simulink model "pd_control"  (R2023b)
settings: Solver=VariableStepAuto  StartTime=0.0  StopTime=10.0  RelTol=1e-3
values from neighbouring files (symbols this model uses):
  a = [x;y;z]    [generate_trajectory.m]    (also in init.m = 1)
  A = 0.1    [generate_trajectory.m]    (also in get_FrictionTorque.m = fp(1,:); init.m = 0.4)
  B = 0.1    [generate_trajectory.m]    (also in init.m = 0.4)
  b = 2    [generate_trajectory.m]    (also in init.m)
  d = pi/2    (= 1.57079632679)    [init.m]
  dq0 = [0.0 ; 0.0; 0.0 ; 0.0; 0.0 ; 0.0; 0.0]    [init.m]
  Kp = 10*eye(7)    [init.m]
  Kv = 10*eye(7)    [init.m]
  Lambda_IK = 10*eye(3)    [init.m]
  lev_mar = false    [init.m]
  mu_0 = 1e-2    (= 0.01)    [init.m]
  p0 = [0.85; 0.85; 0.85]    [init.m]
  q0 = [0 0 0 0 0 0 0]    [FRANKA_model.m]    (also in generate_trajectory.m = [0 pi/3 0 pi/6 0 0 0]; init.m = [0.25 ; 0.25; 0.25 ; 0.25; 0.25 ; 0.25; 0.25])
  rel_err = 0.0    (= 0)    [init.m]
libraries: robotmaniplib x1
settings Model: Creator=franc  LastModifiedBy=franc

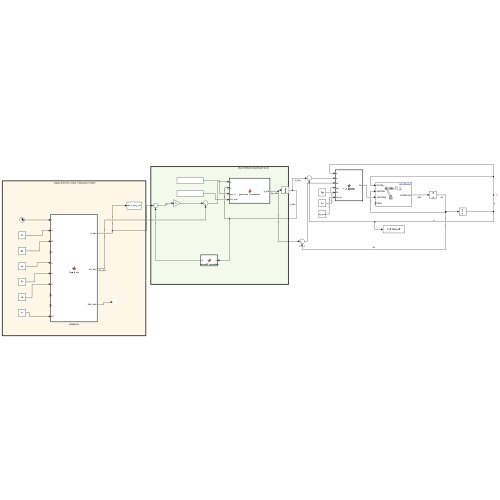
[thumbnail: Simulink's stored preview of the top-level diagram]
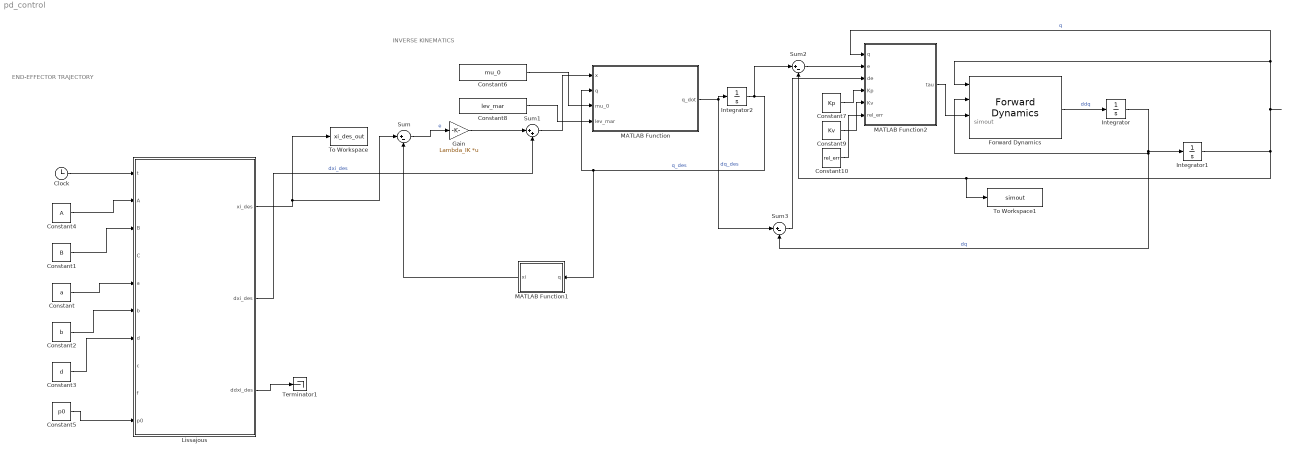
== system pd_control ==
  note: simout
  note: END-EFFECTOR TRAJECTORY
  note: INVERSE KINEMATICS
  Clock : Clock
  Constant : Constant  Value=a
  Constant1 : Constant  Value=B
  Constant10 : Constant  Value=rel_err
  Constant2 : Constant  Value=b
  Constant3 : Constant  Value=d
  Constant4 : Constant  Value=A
  Constant5 : Constant  Value=p0
  Constant6 : Constant  Value=mu_0
  Constant7 : Constant  Value=Kp  VectorParams1D=off
  Constant8 : Constant  Value=lev_mar
  Constant9 : Constant  Value=Kv  VectorParams1D=off
  Forward Dynamics : robotmaniplib/Forward Dynamics  RigidBodyTree=robotModel  SimulateUsing=Interpreted execution
  Gain : Gain  Gain=Lambda_IK  Multiplication=Matrix(K*u)
  Integrator : Integrator  InitialCondition=dq0
  Integrator1 : Integrator  InitialCondition=q0
  Integrator2 : Integrator  InitialCondition=q0
  Lissajous : MATLAB Function  TreatAsAtomicUnit=on
  MATLAB Function : MATLAB Function  TreatAsAtomicUnit=on
  MATLAB Function1 : MATLAB Function  TreatAsAtomicUnit=on
  MATLAB Function2 : MATLAB Function  TreatAsAtomicUnit=on
  Sum : Sum  Inputs=|+-
  Sum1 : Sum  Inputs=|++
  Sum2 : Sum  Inputs=|+-
  Sum3 : Sum  Inputs=|+-
  Terminator1 : Terminator
  To Workspace : ToWorkspace  VariableName=xi_des_out  SaveFormat=Timeseries  SampleTime=-1
  To Workspace1 : ToWorkspace  VariableName=simout  SaveFormat=Timeseries  SampleTime=-1
  wires:
  Forward Dynamics/1 -> Integrator/1  "ddq"
  Integrator/1 -> Sum3/2, Forward Dynamics/2, Integrator1/1  "dq"
  Integrator1/1 -> MATLAB Function2/1(q), Forward Dynamics/1, To Workspace1/1, Sum2/2  "q"
  MATLAB Function/1(q_dot) -> Integrator2/1, Sum3/1  "dq_des"
  Integrator2/1 -> Sum2/1, MATLAB Function1/1(q), MATLAB Function/2(q)  "q_des"
  Constant3/1 -> Lissajous/7(d)
  Constant5/1 -> Lissajous/10(p0)
  Lissajous/1(xi_des) -> To Workspace/1, Sum/1
  Clock/1 -> Lissajous/1(t)
  Constant4/1 -> Lissajous/2(A)
  Constant/1 -> Lissajous/5(a)
  Constant1/1 -> Lissajous/3(B)
  Constant2/1 -> Lissajous/6(b)
  Lissajous/3(ddxi_des) -> Terminator1/1
  MATLAB Function1/1(xi) -> Sum/2
  Gain/1 -> Sum1/1
  Sum/1 -> Gain/1  "e"
  Sum1/1 -> MATLAB Function/1(x)
  Constant6/1 -> MATLAB Function/3(mu_0)
  Constant8/1 -> MATLAB Function/4(lev_mar)
  Lissajous/2(dxi_des) -> Sum1/2  "dxi_des"
  Sum2/1 -> MATLAB Function2/2(e)
  Sum3/1 -> MATLAB Function2/3(de)
  Constant7/1 -> MATLAB Function2/4(Kp)
  Constant9/1 -> MATLAB Function2/5(Kv)
  MATLAB Function2/1(tau) -> Forward Dynamics/3
  Constant10/1 -> MATLAB Function2/6(rel_err)

== matlab function pd_control/MATLAB Function1 ==
  data: q input; xi output
function xi = forwardKinematics(q)
q1 = q(1);
q2 = q(2);
q3 = q(3);
q4 = q(4);
q5 = q(5);
q6 = q(6);
q7 = q(7);
T01r = [cos(q1), -sin(q1), 0;
       sin(q1) , cos(q1), 0;
        0, 0, 1];
T12r = [cos(q2), -sin(q2), 0;
       sin(q2) , cos(q2), 0;
        0, 0, 1] * [1, 0, 0;
            0, cos(-pi/2), -sin(-pi/2);
            0, sin(-pi/2), cos(-pi/2)]; 
T23r = [cos(q3), -sin(q3), 0;
       sin(q3) , cos(q3), 0;
        0, 0, 1] * [1, 0, 0;
            0, cos(pi/2), -sin(pi/2);
            0, sin(pi/2), cos(pi/2)]; 

T23t = [0 0 0.42]';


T34r = [cos(q4), -sin(q4), 0;
       sin(q4) , cos(q4), 0;
        0, 0, 1] * [1, 0, 0;
            0, cos(pi/2), -sin(pi/2);
            0, sin(pi/2), cos(pi/2)]; 
T45r = [cos(q5), -sin(q5), 0;
       sin(q5) , cos(q5), 0;
        0, 0, 1] * [1, 0, 0;
            0, cos(-pi/2), -sin(-pi/2);
            0, sin(-pi/2), cos(-pi/2)]; 
T45t = [0 0 0.4]';

T56r = [cos(q6), -sin(q6), 0;
       sin(q6) , cos(q6), 0;
        0, 0, 1] * [1, 0, 0;
            0, cos(-pi/2), -sin(-pi/2);
            0, sin(-pi/2), cos(-pi/2)]; 
T67r = [cos(q7), -sin(q7), 0;
       sin(q7) , cos(q7), 0;
        0, 0, 1] * [1, 0, 0;
            0, cos(pi/2), -sin(pi/2);
            0, sin(pi/2), cos(pi/2)]; 

O33 = zeros(1,3);

    T =[T01r, O33';
    O33, 1]*[T12r, O33';
    O33, 1]*[T23r, T23t;
    O33, 1]*[T34r, O33';
    O33, 1]*[T45r, T45t;
    O33,1]*[T56r,  O33';
    O33, 1]*[T67r, O33';
    O33, 1];


xi = T(1:3,4);

== matlab function pd_control/MATLAB Function ==
  data: x input; q_dot output size=7; q input; mu_0 input; lev_mar input
function q_dot = jacobian_inversion(x, q, mu_0, lev_mar)
    
    % Getting jacobian and forward kinematics for current guess
    J = get_geometric_Jacobian(q);
    
    % Jacobian inversion
    J_star = zeros(size(J(1:3,:).')); % preallocating
    if lev_mar
        J_star = inv(J(1:3,:).'*J(1:3,:) + mu_0*diag(diag(J(1:3,:).'*J(1:3,:))))*J(1:3,:).';
    else
        J_star = inv(J(1:3,:));
    end
    
q_dot = J_star * x;

== matlab function pd_control/Lissajous ==
  data: t input; xi_des output; A input; B input; C input; a input; b input; d input; c input; f input; dxi_des output; ddxi_des output; p0 input
function [xi_des, dxi_des, ddxi_des] = lissajous(t,A,B,C,a,b,d,c,f,p0)

xi_des = [A*sin(t); B*sin(b*t+d); C*sin(c*t+f)] + p0;
dxi_des = [A*cos(t); B*b*cos(b*t+d); C*c*cos(c*t+f)]
ddxi_des = [-A*sin(t); -B*b^2*sin(b*t+d); -C*c^2*sin(c*t+f)]

== matlab function pd_control/MATLAB Function2 ==
  data: q input; tau output; e input; de input; Kp input; Kv input; rel_err input
function tau = PD_control(q, e, de, Kp, Kv, rel_err)
   
    G = get_gravity_matrix(q);
    % Adding uncertainty
    G = G.*(1 + rel_err);
    
   
    tau = Kv*de + Kp*e + G;
    
end
